simulink model "quad2LQR"  (R2020a)
settings: Solver=FixedStepAuto  StartTime=0.0  StopTime=trajeto_arena.t(end)  FixedStep=0.001  RelTol=1e-3
values from neighbouring files (symbols this model uses):
  A = zeros(12)    [controlador.m]
  B = zeros(12,4)    [controlador.m]
  C = eye(12)    [controlador.m]
  D = zeros(12,4)    [controlador.m]
  K = lqr(A,B,Q,R)    [controlador.m]
  psi_spline = (pi - tan)    [trajeto.m]
  x_spline = pchip(t_ref,x_ref,t_spline)    [trajeto.m]
  y_spline = pchip(t_ref,y_ref,t_spline)    [trajeto.m]
  z_spline = pchip(t_ref,z_ref,t_spline)    [trajeto.m]
undefined symbols (not defined in the file or in its folder): quad
libraries: vrlib x1
settings Model: Creator=aless  LastModifiedBy=aless

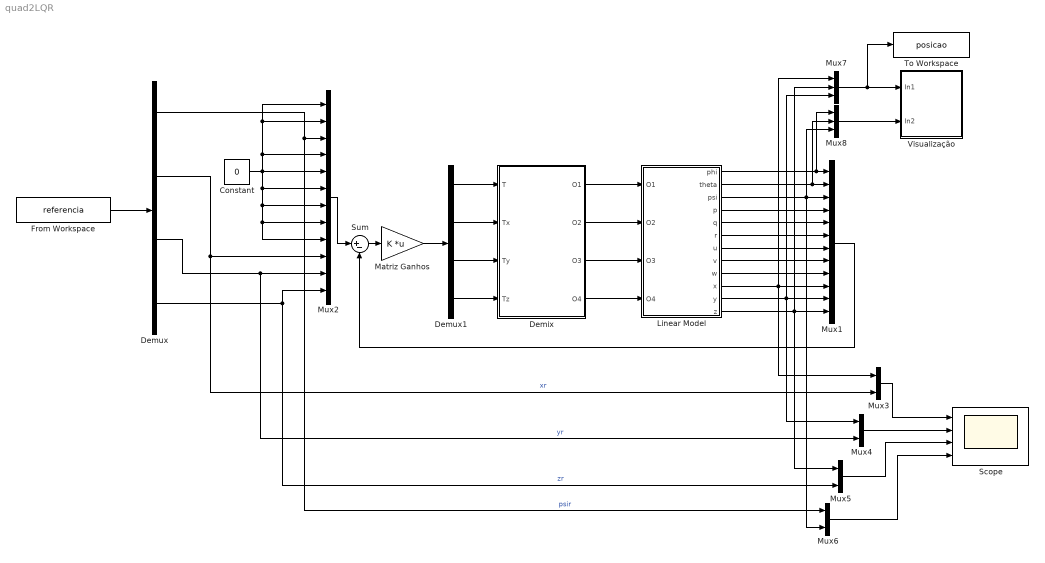
== system quad2LQR ==
  Constant : Constant  Value=0
  Demix : Subsystem
  Demux : Demux
  Demux1 : Demux
  From Workspace : FromWorkspace  VariableName=referencia
  Linear Model : Subsystem
  Matriz Ganhos : Gain  Gain=K  Multiplication=Matrix(K*u)
  Mux1 : Mux  Inputs=12
  Mux2 : Mux  Inputs=12
  Mux{3..6} (4 alike) : Mux  Inputs=2
  Mux7 : Mux  Inputs=3
  Mux8 : Mux  Inputs=3
  Scope : Scope  NumInputPorts=4
  Sum : Sum  Inputs=|+-
  To Workspace : ToWorkspace  VariableName=posicao  SaveFormat=Timeseries  SampleTime=-1
  Visualização : Subsystem
  wires:
  Demix/1(O1) -> Linear Model/1(O1)
  Demix/3(O3) -> Linear Model/3(O3)
  Demix/2(O2) -> Linear Model/2(O2)
  Demix/4(O4) -> Linear Model/4(O4)
  From Workspace/1 -> Demux/1
  Mux2/1 -> Sum/1
  Sum/1 -> Matriz Ganhos/1
  Demux/1 -> Mux2/3, Mux6/1  "psir"
  Demux/2 -> Mux3/2, Mux2/10  "xr"
  Demux/3 -> Mux4/2, Mux2/11  "yr"
  Demux/4 -> Mux2/12, Mux5/2  "zr"
  Constant/1 -> Mux2/5, Mux2/6, Mux2/7, Mux2/8, Mux2/9, Mux2/4, Mux2/2, Mux2/1
  Matriz Ganhos/1 -> Demux1/1
  Demux1/1 -> Demix/1(T)
  Demux1/4 -> Demix/4(Tz)
  Mux3/1 -> Scope/1
  Mux5/1 -> Scope/3
  Mux4/1 -> Scope/2
  Demux1/2 -> Demix/2(Tx)
  Demux1/3 -> Demix/3(Ty)
  Mux6/1 -> Scope/4
  Mux7/1 -> To Workspace/1, Visualização/1(In1)
  Mux8/1 -> Visualização/2(In2)
  Linear Model/1(phi) -> Mux8/1, Mux1/1
  Linear Model/2(theta) -> Mux8/2, Mux1/2
  Linear Model/3(psi) -> Mux6/2, Mux8/3, Mux1/3
  Linear Model/4(p) -> Mux1/4
  Linear Model/5(q) -> Mux1/5
  Linear Model/6(r) -> Mux1/6
  Linear Model/7(u) -> Mux1/7
  Linear Model/8(v) -> Mux1/8
  Linear Model/9(w) -> Mux1/9
  Linear Model/10(x) -> Mux3/1, Mux7/1, Mux1/10
  Linear Model/11(y) -> Mux4/1, Mux7/3, Mux1/11
  Linear Model/12(z) -> Mux5/1, Mux7/2, Mux1/12
  Mux1/1 -> Sum/2

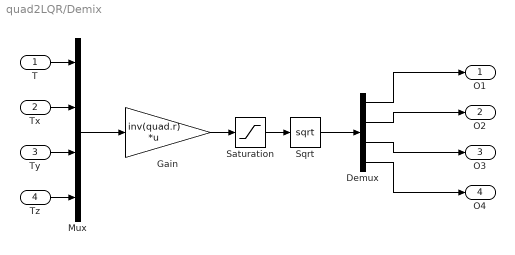
== system quad2LQR/Demix ==
  T : Inport
  Tx : Inport  Port=2
  Ty : Inport  Port=3
  Tz : Inport  Port=4
  Demux : Demux
  Gain : Gain  Gain=inv(quad.r)  Multiplication=Matrix(K*u)
  Mux : Mux
  Saturation : Saturate  UpperLimit=470^2  LowerLimit=0  ZeroCross=off
  Sqrt : Sqrt  SaturateOnIntegerOverflow=on
  O1 : Outport
  O2 : Outport  Port=2
  O3 : Outport  Port=3
  O4 : Outport  Port=4
  wires:
  T/1 -> Mux/1
  Tx/1 -> Mux/2
  Ty/1 -> Mux/3
  Tz/1 -> Mux/4
  Mux/1 -> Gain/1
  Gain/1 -> Saturation/1
  Demux/1 -> O1/1
  Demux/2 -> O2/1
  Demux/3 -> O3/1
  Demux/4 -> O4/1
  Sqrt/1 -> Demux/1
  Saturation/1 -> Sqrt/1

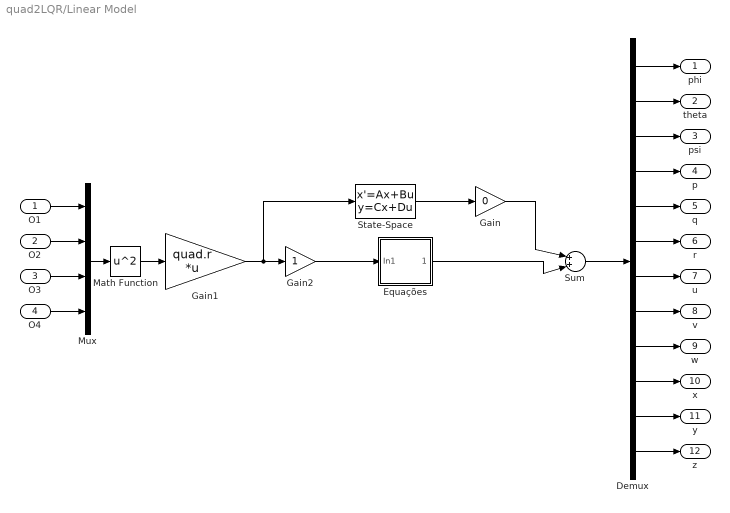
== system quad2LQR/Linear Model ==
  O1 : Inport
  O2 : Inport  Port=2
  O3 : Inport  Port=3
  O4 : Inport  Port=4
  Demux : Demux  Outputs=12
  Equações : Subsystem
  Gain : Gain  Gain=0
  Gain1 : Gain  Gain=quad.r  Multiplication=Matrix(K*u)
  Gain2 : Gain
  Math Function : Math  Operator=square  SaturateOnIntegerOverflow=on
  Mux : Mux
  State-Space : StateSpace  A=A  B=B  C=C  D=D  InitialCondition=0
  Sum : Sum  Inputs=|++|
  phi : Outport
  theta : Outport  Port=2
  psi : Outport  Port=3
  p : Outport  Port=4
  q : Outport  Port=5
  r : Outport  Port=6
  u : Outport  Port=7
  v : Outport  Port=8
  w : Outport  Port=9
  x : Outport  Port=10
  y : Outport  Port=11
  z : Outport  Port=12
  wires:
  O1/1 -> Mux/1
  O4/1 -> Mux/4
  O3/1 -> Mux/3
  O2/1 -> Mux/2
  Mux/1 -> Math Function/1
  Gain1/1 -> State-Space/1, Gain2/1
  Math Function/1 -> Gain1/1
  Gain2/1 -> Equações/1(In1)
  State-Space/1 -> Gain/1
  Equações/1(estado) -> Sum/2
  Sum/1 -> Demux/1
  Demux/1 -> phi/1
  Demux/2 -> theta/1
  Demux/3 -> psi/1
  Demux/4 -> p/1
  Demux/5 -> q/1
  Demux/6 -> r/1
  Demux/7 -> u/1
  Demux/8 -> v/1
  Demux/9 -> w/1
  Demux/10 -> x/1
  Demux/11 -> y/1
  Demux/12 -> z/1
  Gain/1 -> Sum/1

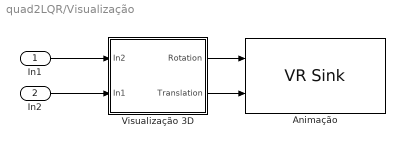
== system quad2LQR/Visualização ==
  In1 : Inport
  In2 : Inport  Port=2
  Animação : vrlib/VR Sink  InstantiateOnLoad=on  SampleTime=0.1  ViewEnable=on  RemoteChange=off  RemoteView=off  FieldsWritten=QuadBody.rotation.4.1.1.double#QuadBody.translation.3.1.1.double  WorldFileName=arena.wrl  WorldDescription=Aerodrome in the Desert  AutoView=on  VideoDimensions=[]  AllowVariableSize=off  FigureProperties="{'Position', 'Name', 'Viewpoint', 'CameraBound', 'CameraDirection', 'CameraPosition', 'CameraUpVector', 'ZoomFactor', 'Antialiasing', 'Headlight', 'Lighting', 'NavPanel', 'Sound', 'StatusBar', 'Stereo3D', 'Stereo3DCameraOffset', 'Stereo3DHIT', 'ToolBar', 'Textures', 'Transparency', 'Triad', 'Wireframe', 'NavZones', 'NavMode', 'NavSpeed', 'CaptureFileFormat', 'CaptureFileName', 'Record2DCompressMethod', 'Record2DCompressQuality', 'Record2D', 'Record2DFileName', 'Record2DFPS'; [1.0000000000000000e+00   7.6000000000000000e+01   1.3660000000000000e+03   6.0100000000000000e+02], 'Aerodrome in the Desert', 'Isometric', 'on', [0.0000000000000000e+00   0.0000000000000000e+00  -1.0000000000000000e+00], [0.0000000000000000e+00   0.0000000000000000e+00   2.0000000000000000e+00], [0.0000000000000000e+00   1.0000000000000000e+00   0.0000000000000000e+00], [1.0000000000000000e+00], 'on', 'on', 'on', 'halfbar', 'on', 'on', 'off', [1.0000000149011612e-01], [0.0000000000000000e+00], 'on', 'on', 'on', 'none', 'off', 'off', 'examine', 'normal', 'tif', '%f_anim_%n.tif', 'auto', [7.5000000000000000e+01], 'off', '%f_anim_%n.avi', 'auto'}"
  Visualização 3D : Subsystem
  wires:
  In1/1 -> Visualização 3D/1(In2)
  In2/1 -> Visualização 3D/2(In1)
  Visualização 3D/2(Translation) -> Animação/2
  Visualização 3D/1(Rotation) -> Animação/1

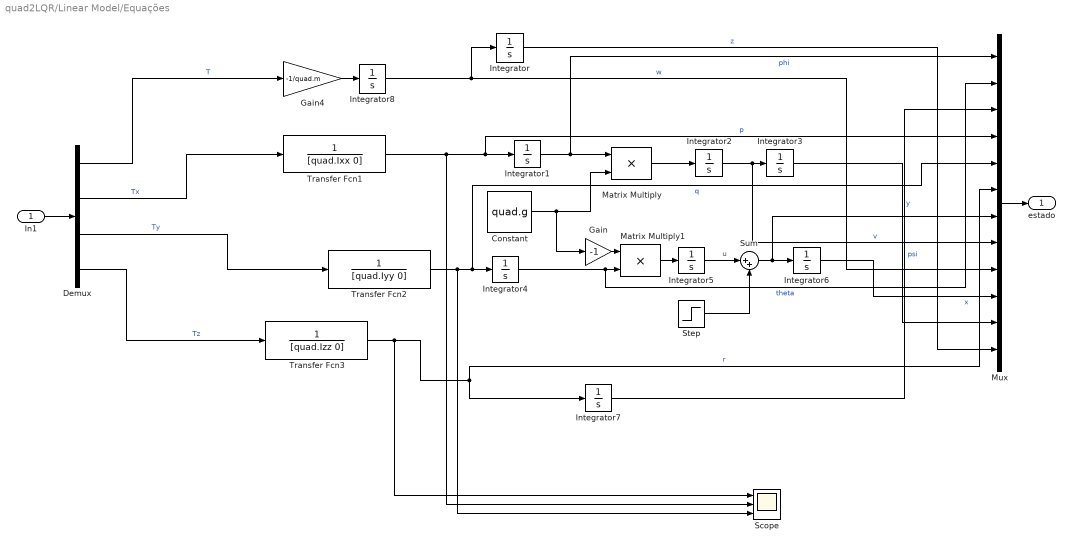
== system quad2LQR/Linear Model/Equações ==
  In1 : Inport
  Constant : Constant  Value=quad.g
  Demux : Demux
  Gain : Gain  Gain=-1
  Gain4 : Gain  Gain=-1/quad.m
  Integrator : Integrator  InitialCondition=z_spline(1)  LimitOutput=on  UpperSaturationLimit=z_spline(1) + 0.01*z_spline(1)  LowerSaturationLimit=z_spline(1) - 0.01*z_spline(1)  WrappedStateUpperValue=0.01  WrappedStateLowerValue=-0.01
  Integrator1 : Integrator  UpperSaturationLimit=0.00261  LowerSaturationLimit=-0.00261
  Integrator2 : Integrator  UpperSaturationLimit=5  LowerSaturationLimit=-5
  Integrator3 : Integrator  InitialCondition=y_spline(1)
  Integrator4 : Integrator  UpperSaturationLimit=0.00261  LowerSaturationLimit=-0.00261
  Integrator5 : Integrator  UpperSaturationLimit=5  LowerSaturationLimit=-5  WrappedStateUpperValue=8  WrappedStateLowerValue=0
  Integrator6 : Integrator  InitialCondition=x_spline(1)
  Integrator7 : Integrator  InitialCondition=psi_spline(1)  LimitOutput=on  UpperSaturationLimit=2*pi  LowerSaturationLimit=0
  Integrator8 : Integrator  InitialCondition=z_spline(1)  UpperSaturationLimit=5  LowerSaturationLimit=-5
  Matrix Multiply : Product
  Matrix Multiply1 : Product
  Mux : Mux  Inputs=12
  Scope : Scope  NumInputPorts=3
  Step : Step  After=5  SampleTime=0
  Sum : Sum  Inputs=|++
  Transfer Fcn1 : TransferFcn  Denominator=[quad.Ixx 0]
  Transfer Fcn2 : TransferFcn  Denominator=[quad.Iyy 0]
  Transfer Fcn3 : TransferFcn  Denominator=[quad.Izz 0]
  estado : Outport
  wires:
  Integrator1/1 -> Mux/1, Matrix Multiply/1  "phi"
  In1/1 -> Demux/1
  Demux/3 -> Transfer Fcn2/1  "Ty"
  Constant/1 -> Matrix Multiply/2, Gain/1
  Integrator8/1 -> Integrator/1, Mux/9  "w"
  Demux/4 -> Transfer Fcn3/1  "Tz"
  Gain/1 -> Matrix Multiply1/1
  Demux/1 -> Gain4/1  "T"
  Matrix Multiply/1 -> Integrator2/1
  Transfer Fcn1/1 -> Scope/2, Mux/4, Integrator1/1  "p"
  Integrator7/1 -> Mux/3  "psi"
  Gain4/1 -> Integrator8/1
  Demux/2 -> Transfer Fcn1/1  "Tx"
  Integrator2/1 -> Mux/8, Integrator3/1  "v"
  Integrator3/1 -> Mux/11  "y"
  Transfer Fcn3/1 -> Scope/1, Integrator7/1, Mux/6  "r"
  Matrix Multiply1/1 -> Integrator5/1
  Integrator4/1 -> Mux/2, Matrix Multiply1/2  "theta"
  Transfer Fcn2/1 -> Scope/3, Mux/5, Integrator4/1  "q"
  Integrator/1 -> Mux/12  "z"
  Integrator6/1 -> Mux/10  "x"
  Mux/1 -> estado/1
  Step/1 -> Sum/2
  Sum/1 -> Mux/7, Integrator6/1
  Integrator5/1 -> Sum/1  "u"

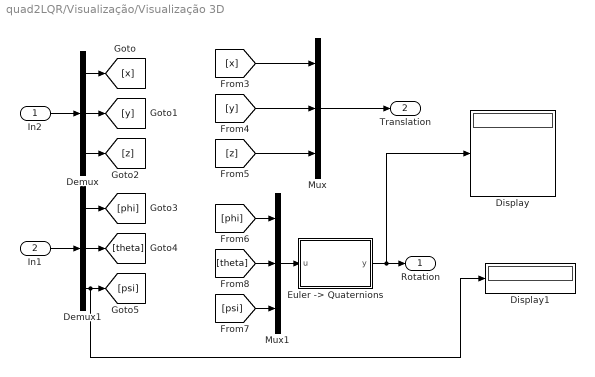
== system quad2LQR/Visualização/Visualização 3D ==
  In2 : Inport
  In1 : Inport  Port=2
  " Euler -> Quaternions" : MATLAB Function  TreatAsAtomicUnit=on
  Demux : Demux  Outputs=3
  Demux1 : Demux  Outputs=3
  Display : Display
  Display1 : Display
  Mux : Mux  Inputs=3
  Mux1 : Mux  Inputs=3
  Rotation : Outport
  Translation : Outport  Port=2
  wires:
  Demux/1 -> [x]
  Demux/2 -> [y]
  In2/1 -> Demux/1
  Demux/3 -> [z]
  In1/1 -> Demux1/1
  Demux1/2 -> [theta]
  Demux1/1 -> [phi]
  Demux1/3 -> Display1/1, [psi]
  [z] -> Mux/3
  [y] -> Mux/2
  [x] -> Mux/1
  [phi] -> Mux1/1
  [theta] -> Mux1/2
  [psi] -> Mux1/3
  Mux/1 -> Translation/1
  Mux1/1 -> " Euler -> Quaternions"/1(u)
  " Euler -> Quaternions"/1(y) -> Display/1, Rotation/1

== matlab function quad2LQR/Visualização/Visualização 3D/ Euler -> Quaternions ==
  data: u input; y output
function y = fcn(u)
y=eul2quat(u')';
end
